simulink model "Observer_particle_reduced"  (R2016a)
settings: Solver=ode4  StartTime=0.0  StopTime=6  FixedStep=0.0001  RelTol=1e-3
settings Model: Creator=DR_C  LastModifiedBy=DR_C
settings DataIOCC: LimitDataPoints=on
settings DebuggingCC: AllowSymbolicDim=off
settings ModelReferenceCC: PropagateSignalLabelsOutOfModel=off
settings GRTTargetCC: GeneratePreprocessorConditionals=Use local settings

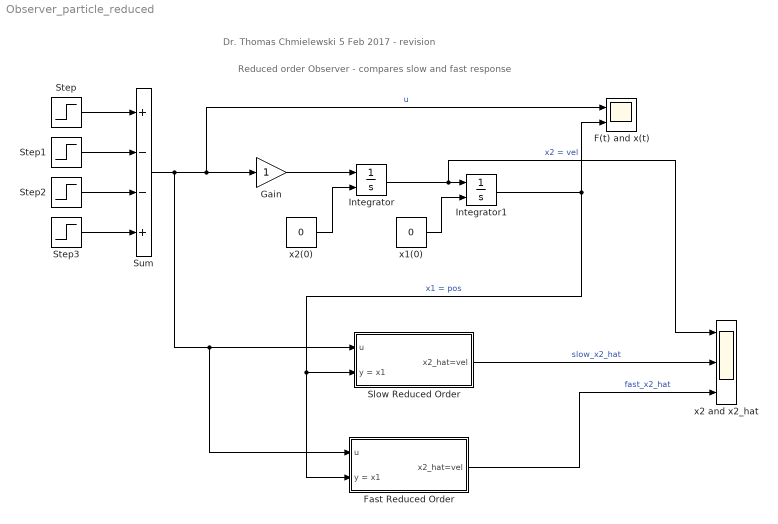
== system Observer_particle_reduced ==
  note: Reduced order Observer - compares slow and fast response
  note: Dr. Thomas Chmielewski 5 Feb 2017 - revision
  F(t) and x(t) : Scope  NumInputPorts=2
  "Fast Reduced Order " : Subsystem
  Gain : Gain
  Integrator : Integrator  InitialConditionSource=external
  Integrator1 : Integrator  InitialConditionSource=external
  "Slow Reduced Order " : Subsystem
  Step : Step  Time=0  SampleTime=0
  Step1 : Step  SampleTime=0
  Step2 : Step  Time=3  SampleTime=0
  Step3 : Step  Time=4  SampleTime=0
  Sum : Sum  Inputs=+--+
  x1(0) : Constant  Value=0
  x2 and x2_hat : Scope  NumInputPorts=3
  x2(0) : Constant  Value=0
  wires:
  Gain/1 -> Integrator/1
  Integrator/1 -> x2 and x2_hat/1, Integrator1/1  "x2 = vel"
  Sum/1 -> "Slow Reduced Order "/1(u), "Fast Reduced Order "/1(u), F(t) and x(t)/1, Gain/1  "u"
  Step3/1 -> Sum/4
  Step2/1 -> Sum/3
  Step1/1 -> Sum/2
  Step/1 -> Sum/1
  Integrator1/1 -> "Slow Reduced Order "/2(y = x1), "Fast Reduced Order "/2(y = x1), F(t) and x(t)/2  "x1 = pos"
  x2(0)/1 -> Integrator/2
  x1(0)/1 -> Integrator1/2
  "Fast Reduced Order "/1(x2_hat=vel) -> x2 and x2_hat/3  "fast_x2_hat"
  "Slow Reduced Order "/1(x2_hat=vel) -> x2 and x2_hat/2  "slow_x2_hat"

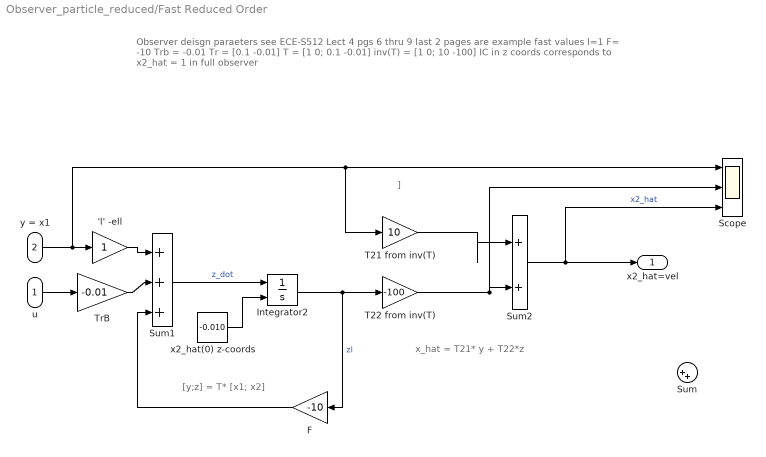
== system Observer_particle_reduced/Fast Reduced Order  ==
  note: [y;z] = T* [x1; x2]
  note: x_hat = T21* y + T22*z
  note: Observer deisgn paraeters see ECE-S512 Lect 4 pgs 6 thru 9 last 2 pages are example
      | fast values
      |
      | l=1 F= -10 Trb = -0.01
      | Tr = [0.1 -0.01] T = [1 0; 0.1 -0.01] inv(T) = [1 0; 10 -100]
      | IC in z coords corresponds to x2_hat = 1 in full observer
  note: ]
  u : Inport
  y = x1 : Inport  Port=2
  'l' -ell : Gain
  F : Gain  Gain=-10
  Integrator2 : Integrator  InitialConditionSource=external
  Scope : Scope  NumInputPorts=3
  Sum : Sum  Inputs=|++
  Sum1 : Sum  Inputs=|+++
  Sum2 : Sum  Inputs=|++
  T21 from inv(T) : Gain  Gain=10
  T22 from inv(T) : Gain  Gain=-100
  TrB : Gain  Gain=-0.01
  x2_hat(0) z-coords : Constant  Value=-0.010
  x2_hat=vel : Outport
  wires:
  y = x1/1 -> T21 from inv(T)/1, Scope/1, 'l' -ell/1
  u/1 -> TrB/1
  Integrator2/1 -> F/1, T22 from inv(T)/1  "zl"
  Sum2/1 -> x2_hat=vel/1, Scope/3  "x2_hat"
  F/1 -> Sum1/3
  'l' -ell/1 -> Sum1/1
  x2_hat(0) z-coords/1 -> Integrator2/2
  TrB/1 -> Sum1/2
  Sum1/1 -> Integrator2/1  "z_dot"
  T22 from inv(T)/1 -> Scope/2, Sum2/2
  T21 from inv(T)/1 -> Sum2/1

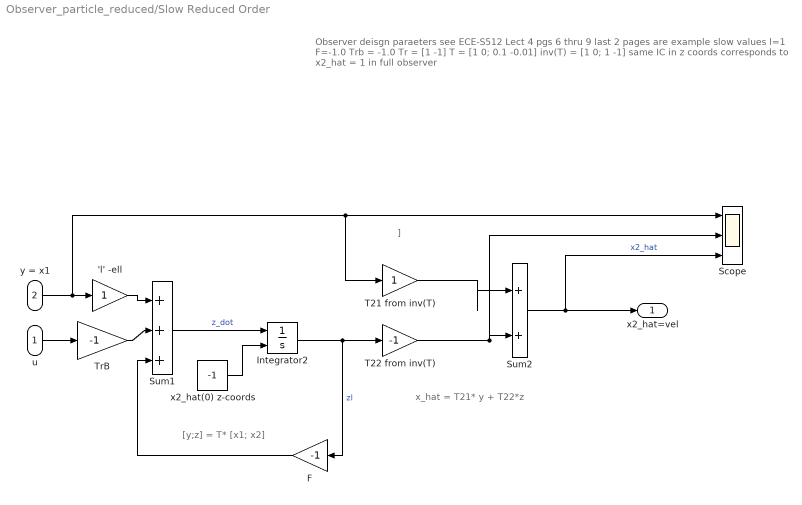
== system Observer_particle_reduced/Slow Reduced Order  ==
  note: [y;z] = T* [x1; x2]
  note: x_hat = T21* y + T22*z
  note: Observer deisgn paraeters see ECE-S512 Lect 4 pgs 6 thru 9 last 2 pages are example
      | slow values
      | l=1 F=-1.0 Trb = -1.0
      | Tr = [1 -1] T = [1 0; 0.1 -0.01] inv(T) = [1 0; 1 -1] same
      | IC in z coords corresponds to x2_hat = 1 in full observer
  note: ]
  u : Inport
  y = x1 : Inport  Port=2
  'l' -ell : Gain
  F : Gain  Gain=-1
  Integrator2 : Integrator  InitialConditionSource=external
  Scope : Scope  NumInputPorts=3
  Sum1 : Sum  Inputs=|+++
  Sum2 : Sum  Inputs=|++
  T21 from inv(T) : Gain
  T22 from inv(T) : Gain  Gain=-1
  TrB : Gain  Gain=-1
  x2_hat(0) z-coords : Constant  Value=-1
  x2_hat=vel : Outport
  wires:
  y = x1/1 -> T21 from inv(T)/1, Scope/1, 'l' -ell/1
  u/1 -> TrB/1
  Integrator2/1 -> F/1, T22 from inv(T)/1  "zl"
  Sum2/1 -> x2_hat=vel/1, Scope/3  "x2_hat"
  F/1 -> Sum1/3
  'l' -ell/1 -> Sum1/1
  x2_hat(0) z-coords/1 -> Integrator2/2
  TrB/1 -> Sum1/2
  Sum1/1 -> Integrator2/1  "z_dot"
  T22 from inv(T)/1 -> Scope/2, Sum2/2
  T21 from inv(T)/1 -> Sum2/1
